simulink model "Galvo_sys_Ccont_Pcont_cc_GUT_v63_adc"  (R2013a)
settings: Solver=ode45  StartTime=0.0  StopTime=5e-3  FixedStep=FS  MaxStep=1e-5  RelTol=1e-3  AbsTol=1e-5
PreLoadFcn:
  | vname=@(x) inputname(1);
  | paramCtrl=evalin('base','paramCtrl;');
  | I_LIM=str2num(paramCtrl.I_LIM);
  | Kbc=str2num(paramCtrl.Kbc);
  | FS=evalin('base','FS;');
InitFcn:
  | %%%%%%  set scope time range
  | T_STOP=str2num(get_param(gcs,'StopTime'));
  | if numel(T_STOP) > 1
  |    T_STOP=T_STOP(2);
  | else
  |    T_STOP=T_STOP(1);
  | end
  | T_STOP=num2str(T_STOP);
  | 
  | %%%%%%  set scope time range in system @init_callback_fct
  | T_STOP=num2str(str2num(get_param(gcs,'StopTime')));
  | 
  | childs = allchild(0);
  | sol=strfind(upper(get(allchild(0),'Tag')),'VIEWER_PARAMETERS');
  | 
  | if iscell(sol)
  |    ind=find(~cellfun(@isempty, strfind(upper(get(allchild(0),'Tag')),'VIEWER_PARAMETERS')));
  | else
  |    ind=sol;
  | end
  | %ind=find(~cellfun(@isempty, {strfind(upper(get(allchild(0),'Tag')),'VIEWER_PARAMETERS'),[]}))
  | if ~isempty(ind)
  |    for k=1:length(childs(ind))
  |       set_param(getfield(get(childs(ind(k)),'UserData'),'block'),'TimeRange',T_STOP);
  |       get_param(getfield(get(childs(ind(k)),'UserData'),'block'),'TimeRange');
  | %    set_param(getfield(get(childs(ind),'UserData'),'block'),'TimeRange',T_STOP);
  | %    get_param(getfield(get(childs(ind),'UserData'),'block'),'TimeRange');
  |    end
  | else
  |     warning(sprintf('VIEWER_PARAMETERS object not found\nOpen the config dialog by hand for the first sim start'))
  | end
StartFcn:
  | I_LIM=str2num(paramCtrl.I_LIM);
  | Kbc=str2num(paramCtrl.Kbc);
  | %FS=evalin('base','FS;');
values from neighbouring files (symbols this model uses):
  FB_EN = 1    [GalvoModel_v6_sys.m]    (also in Galvo_process_analyze.m = k-1; kompl_kreis_linmod_sensitiv.m)
  Lc = 170e-6    (= 0.00017)    [GalvoModel_v6_sys.m]    (also in Galvo_process_analyze.m)
  Rc = 1.5    [GalvoModel_v6_sys.m]    (also in Galvo_process_analyze.m; frequenzgang_nichtinvert_opamp_koblitz_eas.m = 1)
  Rsh = 0.003    [GalvoModel_v6_sys.m]    (also in Galvo_sys_proto_v13_OFFSETS_MODEL_PT1B_proc.m = 0.075; frequenzgang_nichtinvert_opamp_koblitz_eas.m = 0.015)
undefined symbols (not defined in the file or in its folder): JR, KBM, KFR, KMT, KTB
libraries: simulink x3, simulink_extras x1, dspsigops x1
settings Model: BufferReuse=off  Creator=mainster  LastModifiedBy=mainster
settings SolverCC: AutoInsertRateTranBlk=on
settings DataIOCC: LimitDataPoints=off  SaveOutput=off  SaveTime=off
settings OptimizationCC: BlockReduction=off  InlineParams=on  OptimizeBlockIOStorage=off  BufferReuse=off  ExpressionFolding=off  LocalBlockOutputs=off
settings DebuggingCC: InitInArrayFormatMsg=none
settings ModelReferenceCC: ModelReferenceNumInstancesAllowed=Single

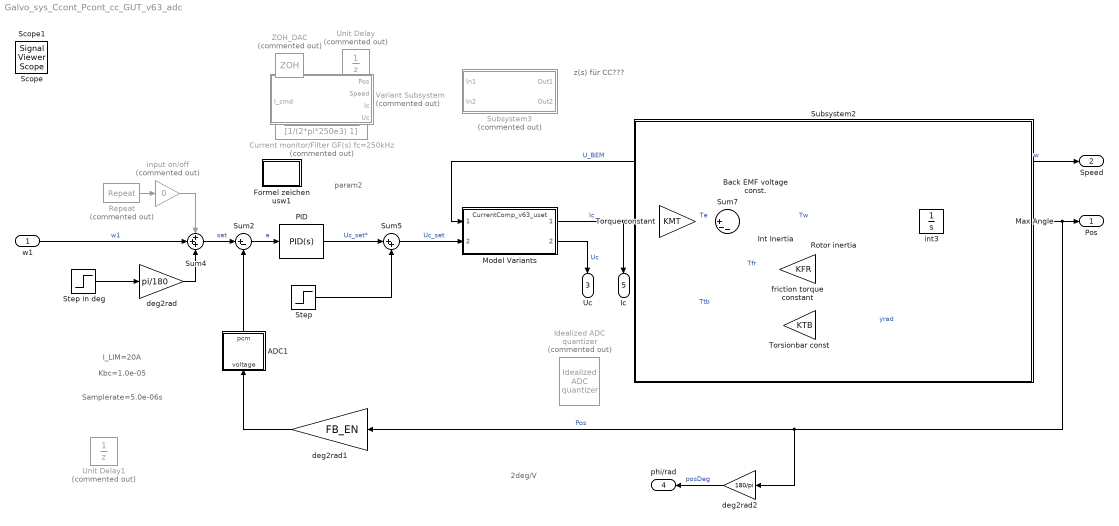
== system Galvo_sys_Ccont_Pcont_cc_GUT_v63_adc ==
  note: 2deg/V
  note: I_LIM=20A
  note: Kbc=1.0e-05
  note: Samplerate=5.0e-06s
  note: z(s) für
      | CC???
  note: param2
  w1 : Inport
  ADC1 : Subsystem  mask{bypass=on}
      mask prompts: bypass "bypass adc"
      mask Callback bypass: %Simulink.Block.eval([gcb '/switch']);
      mask Display:
      | %fprintf('ADC\nGain=%s\n=%i',...
      | %    get_param([gcb '/scale'], 'Gain'),...
      | %    eval( get_param([gcb '/scale'], 'Gain') ));
      | if bypass
      |     color('red')
      |     fprintf('bypass\nADC')
      | else
      |     color('black')
      |     fprintf('ADC')
      | end
  Back EMF voltage const. : Gain  Gain=KBM
  Current monitor/Filter GF(s) fc=250kHz : TransferFcn  Commented=on  Denominator=[1/(2*pi*250e3) 1]
  Formel zeichen usw1 : Subsystem
  Idealized ADC quantizer : simulink_extras/Additional Discrete/Idealized ADC quantizer  Commented=on  NumberOfConverterBits=16  Vmin=-0.5  Vmax=0.5  OutputDataType=int16  OutputNegativeValues=on
  Int Inertia : Integrator
  Max Angle : Saturate  UpperLimit=20*pi/180  LowerLimit=-20*pi/180
      settings: AttributesFormatString=Max=%<UpperLimit>\nMin=%<LowerLimit>
  Model Variants : ModelReference  ModelNameDialog=CurrentComp_v63_uset.slx  SimulationMode=Normal  Variant=on  OverrideUsingVariant=uset  ModelReferenceVersion=1.111  CopyOfModelName=CurrentComp_v63_uset.slx  DefaultDataLogging=on
      settings: AttributesFormatString=%<ActiveVariant>
      mask Display:
      | str=sprintf('%s',get(gcbh,'ModelName'));
      | port_label('input', 2, 'I/U_{Set}','texmode','on')
      | color('red');
      | port_label('input', 1, 'U_{BEM}','texmode','on')
      | color('black');
      | port_label('output', 1, 'I_{Coil}','texmode','on')
      | port_label('output', 2, 'U_{Coil}','texmode','on')
      | %text(.05,.98,['{\fontsize{12}\it\bf' strrep(str,'_',' ') '}'],'horizontalAlignment','left','verticalAlignment','top','texmode','on')
      | text(.5,0.95,['{\fontsize{12}\it\bfG_{cc}(s)}'],'horizontalAlignment','center','verticalAlignment','top','texmode','on')
      | %text(.15,.05,['{\fontsize{10}\itmechanics}'],'horizontalAlignment','left','verticalAlignment','bottom','texmode','on')
  PID : simulink/Continuous/PID Controller  Controller=PID  TimeDomain=Continuous-time  SampleTime=-1  IntegratorMethod=Forward Euler  FilterMethod=Forward Euler  Form=Ideal  P=4.73881789047526  I=18.337628571379  D=0.00402387978016922  N=4838.89581232345  InitialConditionSource=internal  InitialConditionForIntegrator=0  InitialConditionForFilter=0  ExternalReset=none  IgnoreLimit=on  LimitOutput=on  UpperSaturationLimit=30  LowerSaturationLimit=-30  LinearizeAsGain=off  AntiWindupMode=clamping  Kb=0.1  TrackingMode=off  Kt=0  PParamMin=[]  PParamMax=[]  IParamMin=[]  IParamMax=[]  DParamMin=[]  DParamMax=[]  NParamMin=[]  NParamMax=[]  KbParamMin=[]  KbParamMax=[]  KtParamMin=[]  KtParamMax=[]  POutMin=[]  POutMax=[]  IOutMin=[]  IOutMax=[]  DOutMin=[]  DOutMax=[]  NOutMin=[]  NOutMax=[]  KbOutMin=[]  KbOutMax=[]  KtOutMin=[]  KtOutMax=[]  IntegratorOutMin=[]  IntegratorOutMax=[]  FilterOutMin=[]  FilterOutMax=[]  SumOutMin=[]  SumOutMax=[]  SumI1OutMin=[]  SumI1OutMax=[]  SumI2OutMin=[]  SumI2OutMax=[]  SumI3OutMin=[]  SumI3OutMax=[]  SumDOutMin=[]  SumDOutMax=[]  SaturationOutMin=[]  SaturationOutMax=[]  IntegratorContinuousStateAttributes=''  IntegratorStateMustResolveToSignalObject=off  IntegratorRTWStateStorageClass=Auto  FilterContinuousStateAttributes=''  FilterStateMustResolveToSignalObject=off  FilterRTWStateStorageClass=Auto
  Repeat : dspsigops/Repeat  Commented=on  N=length(str2num(get_param([gcs '/Sequence Stair'], 'OutValues')))  InputProcessing=Columns as channels (frame based)  RateOptions=Allow multirate processing  ic=0  mode=Unused parameter value
  Rotor inertia : Gain  Gain=1/JR
  Step : Step  Time=100e-3  SampleTime=0
      settings: AttributesFormatString=Ampl.: %<After>\ntime:%<Time>
  Step in deg : Step  Time=1e-3  After=5  SampleTime=0  ZeroCross=off
      settings: AttributesFormatString=Ampl.: %<After>\ntime:%<Time>
  Subsystem2 : Subsystem
      mask Display: text(.05,.05,['{\fontsize{13}\it\bfGalvo mechanic}'],'horizontalAlignment','left','verticalAlignment','bottom','texmode','on')
  Subsystem3 : Subsystem  Commented=on
  Sum2 : Sum  Inputs=|+-
  Sum4 : Sum  Inputs=+++
  Sum5 : Sum  Inputs=|++
  Sum7 : Sum  Inputs=||+--
  Torque constant : Gain  Gain=KMT
  Torsionbar const : Gain  Gain=KTB
  Unit Delay : UnitDelay  Commented=on  SampleTime=-1
  Unit Delay1 : UnitDelay  Commented=on  SampleTime=-1
  Variant Subsystem : Subsystem  Commented=on  Variant=on  OverrideUsingVariant=Gv_CCsep
  ZOH_DAC : ZeroOrderHold  Commented=on
  deg2rad : Gain  Gain=pi/180
  deg2rad1 : Gain  Gain=FB_EN
  deg2rad2 : Gain  Gain=180/pi
  friction torque constant : Gain  Gain=KFR
  input on/off : Gain  Commented=on  Gain=0  SampleTime=FS
  int3 : Integrator
  Pos : Outport
  Speed : Outport  Port=2
  Uc : Outport  Port=3
  phi/rad : Outport  Port=4
  Ic : Outport  Port=5
  Scope : SignalViewerScope  IOType=viewer  NumInputPorts=5  LegendLocations=|  RefreshTime=0.033391
      | 0.80511      0.9394     0.12993    0.020986
      |       0           0           0           0
      |       0           0           0           0
      |       0           0           0           0
      |       0           0           0           0
      settings: ShowLegends=on  TimeRange=0.02  YMin=-0.02~-0.5~-0.5~-2~-2  YMax=0.1~2~1.5~10~6
  Scope1 : SignalViewerScope  IOType=viewer  NumInputPorts=5  LegendLocations=|  RefreshTime=0.035000
      | 0.81147     0.93803     0.12202    0.021097
      | 0.80046     0.74921     0.13303    0.021097
      | 0.81147     0.55934     0.12202    0.021097
      |       0           0           0           0
      |       0           0           0           0
      settings: ShowLegends=on  TimeRange=0.005  YMin=-5~-5~-5~-5~-5  YMax=5~5~5~5~5
  wires:
  w1/1 -> Sum4/2  "w1"
  Repeat/1 -> input on/off/1
  Sum2/1 -> PID/1  "e"
  Sum4/1 -> Sum2/1  "set"
  Step in deg/1 -> deg2rad/1
  input on/off/1 -> Sum4/1
  deg2rad/1 -> Sum4/3
  Step/1 -> Sum5/2
  int3/1 -> Max Angle/1, Torsionbar const/1  "yrad"
  Int Inertia/1 -> Rotor inertia/1  "Tw"
  Sum7/1 -> Int Inertia/1
  Rotor inertia/1 -> Speed/1, int3/1, Back EMF voltage const./1, friction torque constant/1  "w"
  friction torque constant/1 -> Sum7/3  "Tfr"
  Max Angle/1 -> deg2rad2/1, deg2rad1/1, Pos/1  "Pos"
  Torque constant/1 -> Sum7/1  "Te"
  Torsionbar const/1 -> Sum7/2  "Ttb"
  PID/1 -> Sum5/1  "Uc_set*"
  Sum5/1 -> Model Variants/2  "Uc_set"
  Model Variants/1 -> Ic/1, Torque constant/1  "Ic"
  Model Variants/2 -> Uc/1  "Uc"
  deg2rad1/1 -> ADC1/1(voltage)
  deg2rad2/1 -> phi/rad/1  "posDeg"
  Back EMF voltage const./1 -> Model Variants/1  "U_BEM"
  ADC1/1(pcm) -> Sum2/2

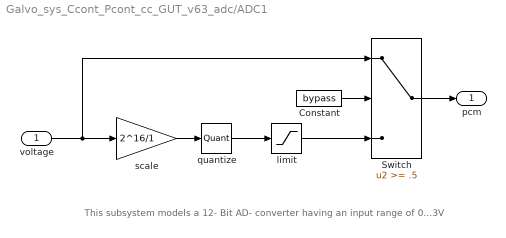
== system Galvo_sys_Ccont_Pcont_cc_GUT_v63_adc/ADC1 ==
  note: This subsystem models a 12- Bit AD- converter
      | having an input  range of 0...3V
  voltage : Inport
  Constant : Constant  Value=bypass
  Switch : Switch  Threshold=.5
  limit : Saturate  UpperLimit=2^15-1  LowerLimit=-2^15
  quantize : Quantizer
  scale : Gain  Gain=2^16/1  SaturateOnIntegerOverflow=on  OutDataTypeStr=Inherit: Same as input  ParamDataTypeStr=Inherit: Same as input
  pcm : Outport
  wires:
  limit/1 -> Switch/3
  scale/1 -> quantize/1
  quantize/1 -> limit/1
  voltage/1 -> Switch/1, scale/1
  Constant/1 -> Switch/2
  Switch/1 -> pcm/1

== system Galvo_sys_Ccont_Pcont_cc_GUT_v63_adc/Formel zeichen usw1 ==
  note: Te: 		electrical torque, gen. by coils		[Nm]
      |  Ic: 			coil current							[A]
      |  Tfr:		rotor dynamic friction torque 		[Nm]
      |  Trb:		torsion bar torque					[Nm]
      |  Tw:		angular momentum				[Nm*s]
      |  w:			angular velocity 					[rad/s]
      |  yrad:		angular position 					[rad]
      |  ydeg:		angular position 					[°]
      |  Ucci:		current controller input				[V]
      |  Ucco:		current controller output			[V]
      |  Ush:		shunt voltage						[V]
  note: L_{c  }	coil inductance 							[H]
      |  R_{c  }	coil resistance							[\Omega]
      |  R_{SH }	current shunt resistance				[\Omega]
      |  J_{R  }	rotor inertia 							[kg*m²]
      |  K_{TB }	torsion bar torque const. 			[Nm/rad]
      |  K_{BM }	back EMF const.							[V*s/rad]
      |  K_{FR }	rotor dyn. friction torque const.	[Nm*s/rad]
      |  K_{MT }	el. magnetic torque const.			[Nm/A]
  note: balance of force: 	Te=Ttb+Tfr
      | 					Te - (Ttb+Tfr)=0  ->  no movement
      |
      |  integrate( 1 Nm )dt = 1 Nm*s
      |  (Nm*s)(kg*m²)⁻¹ = (N*s/kg)*m⁻¹ = m/(s*m) = rad

== system Galvo_sys_Ccont_Pcont_cc_GUT_v63_adc/Subsystem2 ==

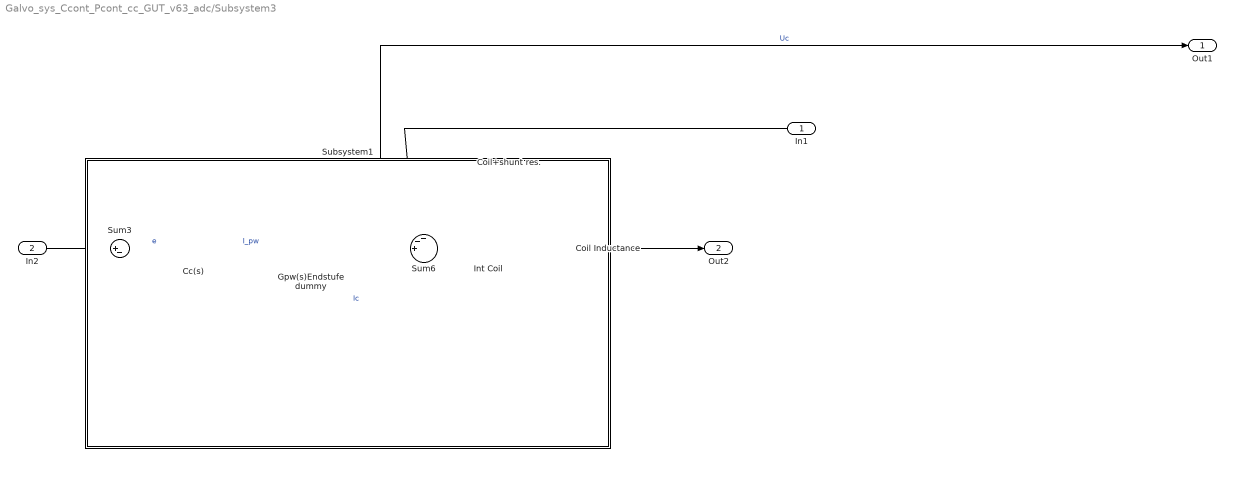
== system Galvo_sys_Ccont_Pcont_cc_GUT_v63_adc/Subsystem3 ==
  In1 : Inport
  In2 : Inport  Port=2
  Cc(s) : simulink/Continuous/PID Controller  Controller=P  TimeDomain=Continuous-time  SampleTime=-1  IntegratorMethod=Forward Euler  FilterMethod=Forward Euler  Form=Ideal  P=59.6963088947406  I=1985.39023021624  D=0  N=100  InitialConditionSource=internal  InitialConditionForIntegrator=0  InitialConditionForFilter=0  ExternalReset=none  LimitOutput=off  UpperSaturationLimit=inf  LowerSaturationLimit=-inf  LinearizeAsGain=on  AntiWindupMode=none  Kb=1  TrackingMode=off  Kt=1  PParamMin=[]  PParamMax=[]  IParamMin=[]  IParamMax=[]  DParamMin=[]  DParamMax=[]  NParamMin=[]  NParamMax=[]  KbParamMin=[]  KbParamMax=[]  KtParamMin=[]  KtParamMax=[]  POutMin=[]  POutMax=[]  IOutMin=[]  IOutMax=[]  DOutMin=[]  DOutMax=[]  NOutMin=[]  NOutMax=[]  KbOutMin=[]  KbOutMax=[]  KtOutMin=[]  KtOutMax=[]  IntegratorOutMin=[]  IntegratorOutMax=[]  FilterOutMin=[]  FilterOutMax=[]  SumOutMin=[]  SumOutMax=[]  SumI1OutMin=[]  SumI1OutMax=[]  SumI2OutMin=[]  SumI2OutMax=[]  SumI3OutMin=[]  SumI3OutMax=[]  SumDOutMin=[]  SumDOutMax=[]  SaturationOutMin=[]  SaturationOutMax=[]  IntegratorContinuousStateAttributes=''  IntegratorStateMustResolveToSignalObject=off  IntegratorRTWStateStorageClass=Auto  FilterContinuousStateAttributes=''  FilterStateMustResolveToSignalObject=off  FilterRTWStateStorageClass=Auto
      settings: AttributesFormatString=P = %<P>
  Coil Inductance : Gain  Gain=1/Lc
  Coil+shunt res. : Gain  Gain=Rc+Rsh
  Gpw(s)Endstufe dummy : Gain
  Int Coil : Integrator
  Subsystem1 : Subsystem
      mask Display: text(.05,.90,['{\fontsize{13}\it\bfCurrent Compensator}'],'horizontalAlignment','left','verticalAlignment','bottom','texmode','on')
  Sum3 : Sum  Inputs=|+-
  Sum6 : Sum  Inputs=--+||
  Out1 : Outport
  Out2 : Outport  Port=2
  wires:
  Int Coil/1 -> Coil Inductance/1
  Coil Inductance/1 -> Out2/1, Sum3/2, Coil+shunt res./1  "Ic"
  Coil+shunt res./1 -> Sum6/1
  Gpw(s)Endstufe dummy/1 -> Out1/1, Sum6/3  "Uc"
  In2/1 -> Sum3/1
  Sum6/1 -> Int Coil/1
  Sum3/1 -> Cc(s)/1  "e"
  Cc(s)/1 -> Gpw(s)Endstufe dummy/1  "I_pw"
  In1/1 -> Sum6/2

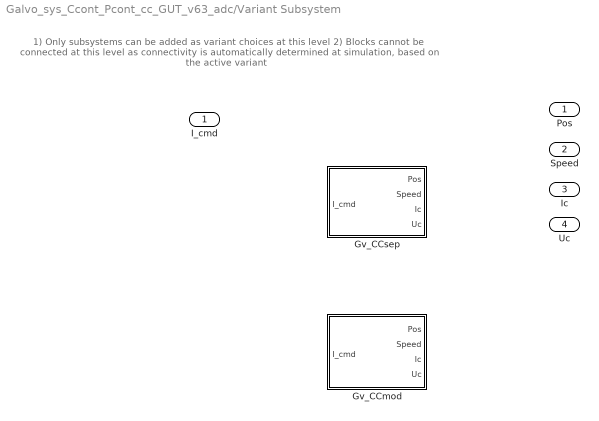
== system Galvo_sys_Ccont_Pcont_cc_GUT_v63_adc/Variant Subsystem ==
  note: 1) Only subsystems can be added as variant choices at this level
      | 2) Blocks cannot be connected at this level as connectivity is
      | automatically determined at simulation, based on the active variant
  I_cmd : Inport
  Gv_CCmod : Subsystem  VariantControl=Gv_CCmod
  Gv_CCsep : Subsystem  VariantControl=Gv_CCsep
  Pos : Outport  SampleTime=FS
  Speed : Outport  Port=2  SampleTime=FS
  Ic : Outport  Port=3  SampleTime=FS
  Uc : Outport  Port=4  SampleTime=FS

== system Galvo_sys_Ccont_Pcont_cc_GUT_v63_adc/Subsystem3/Subsystem1 ==

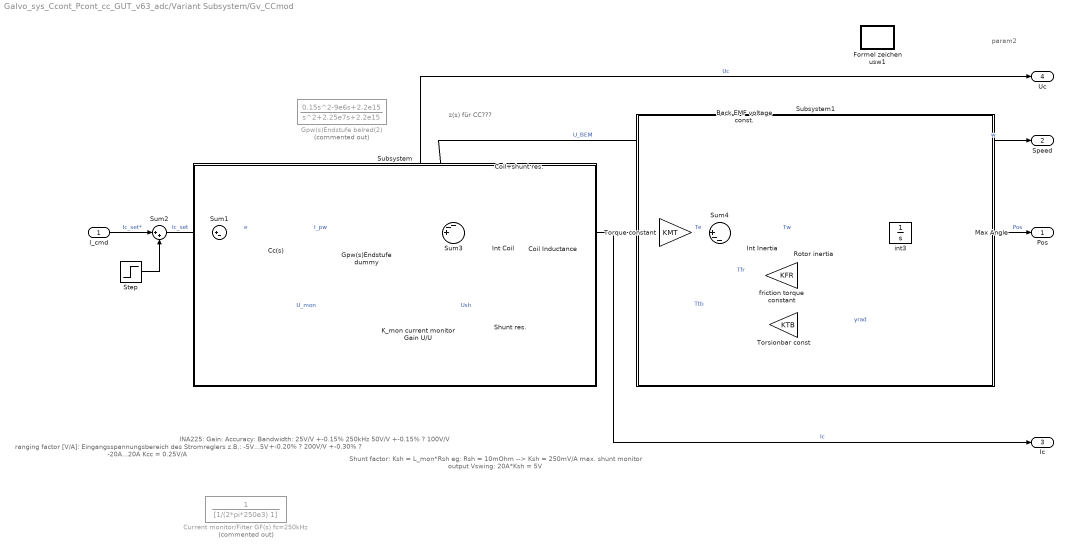
== system Galvo_sys_Ccont_Pcont_cc_GUT_v63_adc/Variant Subsystem/Gv_CCmod ==
  note: z(s) für
      | CC???
  note: ranging factor [V/A]:
      | Eingangsspannungsbereich des
      | Stromreglers z.B.:
      | -5V...5V --> -20A...20A
      | Kcc = 0.25V/A
  note: Shunt factor:
      | Ksh = L_mon*Rsh
      |
      | eg: Rsh = 10mOhm
      |
      | --> Ksh = 250mV/A
      | max. shunt monitor
      | output Vswing:
      | 20A*Ksh = 5V
  note: INA225:
      | Gain:		Accuracy:		Bandwidth:
      | 25V/V		+-0.15%		250kHz
      | 50V/V		+-0.15%		?
      | 100V/V	+-0.20%		?
      | 200V/V	+-0.30%		?
  note: param2
  I_cmd : Inport  SampleTime=FS
  Back EMF voltage const. : Gain  Gain=KBM
  Cc(s) : simulink/Continuous/PID Controller  Controller=P  TimeDomain=Continuous-time  SampleTime=-1  IntegratorMethod=Forward Euler  FilterMethod=Forward Euler  Form=Ideal  P=15.5227390982487  I=1985.39023021624  D=0  N=100  InitialConditionSource=internal  InitialConditionForIntegrator=0  InitialConditionForFilter=0  ExternalReset=none  LimitOutput=off  UpperSaturationLimit=inf  LowerSaturationLimit=-inf  LinearizeAsGain=on  AntiWindupMode=none  Kb=1  TrackingMode=off  Kt=1  PParamMin=[]  PParamMax=[]  IParamMin=[]  IParamMax=[]  DParamMin=[]  DParamMax=[]  NParamMin=[]  NParamMax=[]  KbParamMin=[]  KbParamMax=[]  KtParamMin=[]  KtParamMax=[]  POutMin=[]  POutMax=[]  IOutMin=[]  IOutMax=[]  DOutMin=[]  DOutMax=[]  NOutMin=[]  NOutMax=[]  KbOutMin=[]  KbOutMax=[]  KtOutMin=[]  KtOutMax=[]  IntegratorOutMin=[]  IntegratorOutMax=[]  FilterOutMin=[]  FilterOutMax=[]  SumOutMin=[]  SumOutMax=[]  SumI1OutMin=[]  SumI1OutMax=[]  SumI2OutMin=[]  SumI2OutMax=[]  SumI3OutMin=[]  SumI3OutMax=[]  SumDOutMin=[]  SumDOutMax=[]  SaturationOutMin=[]  SaturationOutMax=[]  IntegratorContinuousStateAttributes=''  IntegratorStateMustResolveToSignalObject=off  IntegratorRTWStateStorageClass=Auto  FilterContinuousStateAttributes=''  FilterStateMustResolveToSignalObject=off  FilterRTWStateStorageClass=Auto
      settings: AttributesFormatString=P = %<P>
  Coil Inductance : Gain  Gain=1/Lc
  Coil+shunt res. : Gain  Gain=Rc+Rsh
  Current monitor/Filter GF(s) fc=250kHz : TransferFcn  Commented=on  Denominator=[1/(2*pi*250e3) 1]
  Formel zeichen usw1 : Subsystem
  Gpw(s)Endstufe balred(2) : TransferFcn  Commented=on  Numerator=[0.15 -9e6 2.2e15]  Denominator=[1 2.25e7 2.2e15]
  Gpw(s)Endstufe dummy : Gain
  Int Coil : Integrator
  Int Inertia : Integrator
  K_mon current monitor Gain U/U : Gain  Gain=1/Rsh
  Max Angle : Saturate  UpperLimit=20*pi/180  LowerLimit=-20*pi/180
      settings: AttributesFormatString=Max=%<UpperLimit>\nMin=%<LowerLimit>
  Rotor inertia : Gain  Gain=1/JR
  Shunt res. : Gain  Gain=Rsh
  Step : Step  Time=0
      settings: AttributesFormatString=%<Time>
  Subsystem : Subsystem
      mask Display: text(.05,.90,['{\fontsize{13}\it\bfCurrent Compensator}'],'horizontalAlignment','left','verticalAlignment','bottom','texmode','on')
  Subsystem1 : Subsystem
      mask Display: text(.05,.05,['{\fontsize{13}\it\bfGalvo mechanic}'],'horizontalAlignment','left','verticalAlignment','bottom','texmode','on')
  Sum1 : Sum  Inputs=|+-
  Sum2 : Sum  Inputs=|++
  Sum3 : Sum  Inputs=--+||
  Sum4 : Sum  Inputs=||+--
  Torque constant : Gain  Gain=KMT
  Torsionbar const : Gain  Gain=KTB
  friction torque constant : Gain  Gain=KFR
  int3 : Integrator
  Pos : Outport  SampleTime=FS
  Speed : Outport  Port=2  SampleTime=FS
  Ic : Outport  Port=3  SampleTime=FS
  Uc : Outport  Port=4  SampleTime=FS
  wires:
  I_cmd/1 -> Sum2/1  "Ic_set*"
  Sum1/1 -> Cc(s)/1  "e"
  Sum3/1 -> Int Coil/1
  Int Coil/1 -> Coil Inductance/1
  Cc(s)/1 -> Gpw(s)Endstufe dummy/1  "I_pw"
  K_mon current monitor Gain U/U/1 -> Sum1/2  "U_mon"
  Shunt res./1 -> K_mon current monitor Gain U/U/1  "Ush"
  Gpw(s)Endstufe dummy/1 -> Uc/1, Sum3/3  "Uc"
  Coil+shunt res./1 -> Sum3/1
  Sum2/1 -> Sum1/1  "Ic_set"
  Step/1 -> Sum2/2
  int3/1 -> Max Angle/1, Torsionbar const/1  "yrad"
  Int Inertia/1 -> Rotor inertia/1  "Tw"
  Sum4/1 -> Int Inertia/1
  Rotor inertia/1 -> Speed/1, int3/1, Back EMF voltage const./1, friction torque constant/1  "w"
  friction torque constant/1 -> Sum4/3  "Tfr"
  Max Angle/1 -> Pos/1  "Pos"
  Coil Inductance/1 -> Ic/1, Torque constant/1, Coil+shunt res./1, Shunt res./1  "Ic"
  Back EMF voltage const./1 -> Sum3/2  "U_BEM"
  Torque constant/1 -> Sum4/1  "Te"
  Torsionbar const/1 -> Sum4/2  "Ttb"

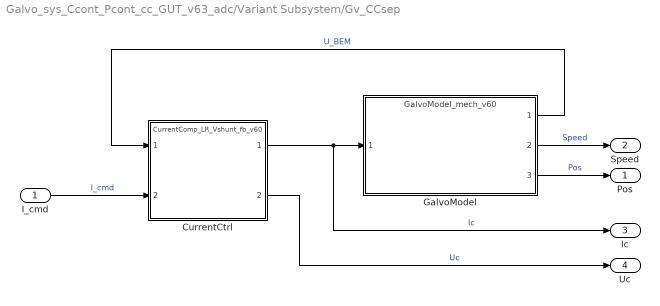
== system Galvo_sys_Ccont_Pcont_cc_GUT_v63_adc/Variant Subsystem/Gv_CCsep ==
  I_cmd : Inport  SampleTime=FS
  CurrentCtrl : ModelReference  ModelNameDialog=CurrentComp_LR_Vshunt_fb_v60.slx  SimulationMode=Normal  Variant=on  OverrideUsingVariant=cc_v20  ModelReferenceVersion=1.94  CopyOfModelName=CurrentComp_LR_Vshunt_fb_v60.slx  DefaultDataLogging=on
      mask Display:
      | str=sprintf('%s',get(gcbh,'ModelName'));
      | port_label('input', 2, 'I_{Set}','texmode','on')
      | color('red');
      | port_label('input', 1, 'U_{BEM}','texmode','on')
      | color('black');
      | port_label('output', 1, 'I_{Coil}','texmode','on')
      | port_label('output', 2, 'U_{Coil}','texmode','on')
      | %text(.05,.98,['{\fontsize{12}\it\bf' strrep(str,'_',' ') '}'],'horizontalAlignment','left','verticalAlignment','top','texmode','on')
      | text(.5,0.95,['{\fontsize{12}\it\bfG_{cc}(s)}'],'horizontalAlignment','center','verticalAlignment','top','texmode','on')
      | %text(.15,.05,['{\fontsize{10}\itmechanics}'],'horizontalAlignment','left','verticalAlignment','bottom','texmode','on')
  GalvoModel : ModelReference  ModelNameDialog=GalvoModel_mech_v60.slx  SimulationMode=Normal  Variant=on  OverrideUsingVariant=v53_neuer_cc  ModelReferenceVersion=1.68  CopyOfModelName=GalvoModel_mech_v60.slx  DefaultDataLogging=on
      mask Display:
      | str=sprintf('%s',get(gcbh,'ModelName'));
      | port_label('input', 1, 'I_{Coil}','texmode','on')
      | color('blue');
      | port_label('output', 3, 'Pos','texmode','on')
      | color('black');
      | port_label('output', 2, 'Speed','texmode','on')
      | port_label('output', 1, 'U_{BEM}','texmode','on')
      | %text(.05,.98,['{\fontsize{12}\it\bf' strrep(str,'_',' ') '}'],'horizontalAlignment','left','verticalAlignment','top','texmode','on')
      | text(.015,.98,['{\fontsize{12}\it\bf' strrep(str,'_','\_') '}'],'horizontalAlignment','left','verticalAlignment','top','texmode','on')
      | text(.15,.05,['{\fontsize{10}\itmechanics}'],'horizontalAlignment','left','verticalAlignment','bottom','texmode','on')
  Pos : Outport  SampleTime=FS
  Speed : Outport  Port=2  SampleTime=FS
  Ic : Outport  Port=3  SampleTime=FS
  Uc : Outport  Port=4  SampleTime=FS
  wires:
  CurrentCtrl/1 -> GalvoModel/1, Ic/1  "Ic"
  GalvoModel/2 -> Speed/1  "Speed"
  GalvoModel/3 -> Pos/1  "Pos"
  GalvoModel/1 -> CurrentCtrl/1  "U_BEM"
  I_cmd/1 -> CurrentCtrl/2  "I_cmd"
  CurrentCtrl/2 -> Uc/1  "Uc"

== system Galvo_sys_Ccont_Pcont_cc_GUT_v63_adc/Variant Subsystem/Gv_CCmod/Formel zeichen usw1 ==
  note: Te: 		electrical torque, gen. by coils		[Nm]
      |  Ic: 			coil current							[A]
      |  Tfr:		rotor dynamic friction torque 		[Nm]
      |  Trb:		torsion bar torque					[Nm]
      |  Tw:		angular momentum				[Nm*s]
      |  w:			angular velocity 					[rad/s]
      |  yrad:		angular position 					[rad]
      |  ydeg:		angular position 					[°]
      |  Ucci:		current controller input				[V]
      |  Ucco:		current controller output			[V]
      |  Ush:		shunt voltage						[V]
  note: L_{c  }	coil inductance 							[H]
      |  R_{c  }	coil resistance							[\Omega]
      |  R_{SH }	current shunt resistance				[\Omega]
      |  J_{R  }	rotor inertia 							[kg*m²]
      |  K_{TB }	torsion bar torque const. 			[Nm/rad]
      |  K_{BM }	back EMF const.							[V*s/rad]
      |  K_{FR }	rotor dyn. friction torque const.	[Nm*s/rad]
      |  K_{MT }	el. magnetic torque const.			[Nm/A]
  note: balance of force: 	Te=Ttb+Tfr
      | 					Te - (Ttb+Tfr)=0  ->  no movement
      |
      |  integrate( 1 Nm )dt = 1 Nm*s
      |  (Nm*s)(kg*m²)⁻¹ = (N*s/kg)*m⁻¹ = m/(s*m) = rad

== system Galvo_sys_Ccont_Pcont_cc_GUT_v63_adc/Variant Subsystem/Gv_CCmod/Subsystem ==

== system Galvo_sys_Ccont_Pcont_cc_GUT_v63_adc/Variant Subsystem/Gv_CCmod/Subsystem1 ==
